simulink model "vtol50kg_linearization"  (R2024b)
settings: Solver=FixedStepAuto  StartTime=0.0  StopTime=10  FixedStep=5/1000  RelTol=1e-3
settings Model: DataDictionary=nextpilot_datadict.sldd  Creator=CETCA  LastModifiedBy=CETCA
settings DataIOCC: ExternalInput=getinputstruct(report8)  InitialState=getstatestruct(report8)  LoadExternalInput=on  LoadInitialState=on

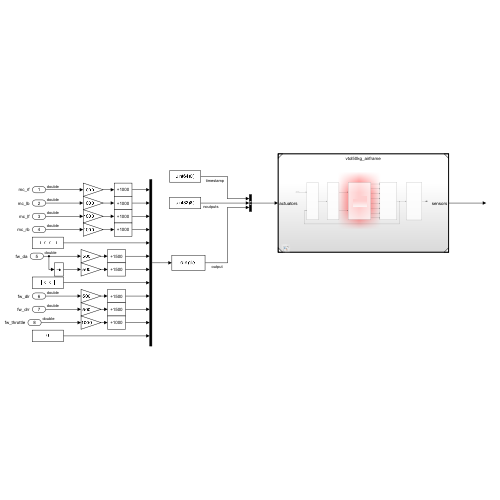
[thumbnail: Simulink's stored preview of the top-level diagram]
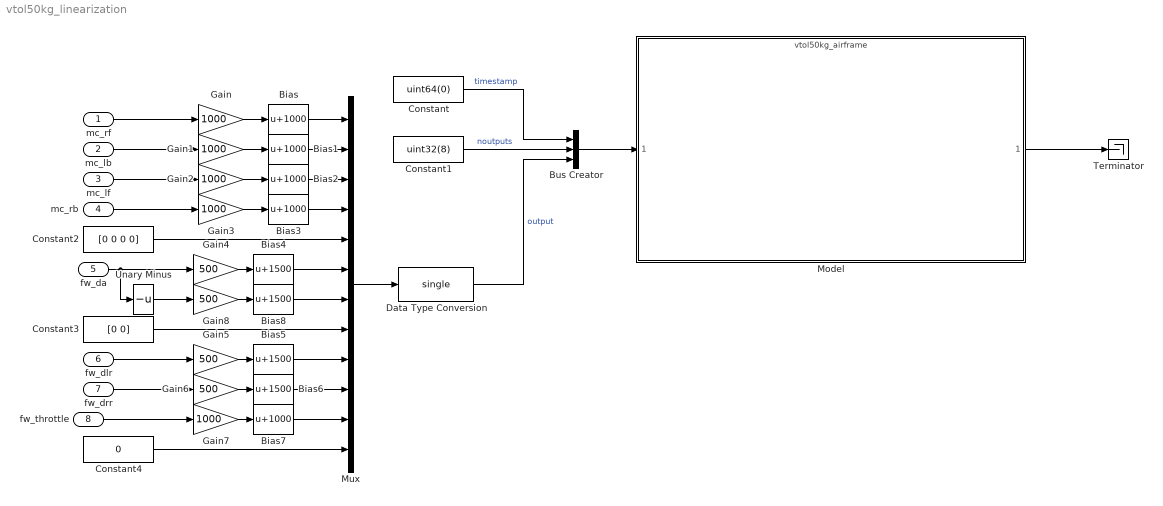
== system vtol50kg_linearization ==
  mc_rf : Inport  OutMin=0  OutMax=1  OutDataTypeStr=double
  mc_lb : Inport  Port=2  OutMin=0  OutMax=1  OutDataTypeStr=double
  mc_lf : Inport  Port=3  OutMin=0  OutMax=1  OutDataTypeStr=double
  mc_rb : Inport  Port=4  OutMin=0  OutMax=1  OutDataTypeStr=double
  fw_da : Inport  Port=5  OutMin=-1  OutMax=1  OutDataTypeStr=double
  fw_dlr : Inport  Port=6  OutMin=-1  OutMax=1  OutDataTypeStr=double
  fw_drr : Inport  Port=7  OutMin=-1  OutMax=1  OutDataTypeStr=double
  fw_throttle : Inport  Port=8  OutMin=0  OutMax=1  OutDataTypeStr=double
  Bias{,1..3,7} (5 alike) : Bias  Bias=1000  SaturateOnIntegerOverflow=off
  Bias{4..6,8} (4 alike) : Bias  Bias=1500  SaturateOnIntegerOverflow=off
  Bus Creator : BusCreator  Inputs=3
  Constant : Constant  Value=uint64(0)
  Constant1 : Constant  Value=uint32(8)
  Constant2 : Constant  Value=[0 0 0 0]
  Constant3 : Constant  Value=[0 0]
  Constant4 : Constant  Value=0
  Data Type Conversion : DataTypeConversion  OutDataTypeStr=single  SaturateOnIntegerOverflow=off  RndMeth=Floor
  Gain{,1..3,7} (5 alike) : Gain  Gain=1000
  Gain{4..6,8} (4 alike) : Gain  Gain=500
  Model : ModelReference  ModelNameDialog=vtol50kg_airframe.slx  SimulationMode=Normal  ModelReferenceVersion=5.112
  Mux : Mux  Inputs=12
  Terminator : Terminator
  Unary Minus : UnaryMinus
  wires:
  Bus Creator/1 -> Model/1
  Constant/1 -> Bus Creator/1  "timestamp"
  Constant1/1 -> Bus Creator/2  "noutputs"
  Mux/1 -> Data Type Conversion/1
  Data Type Conversion/1 -> Bus Creator/3  "output"
  Model/1 -> Terminator/1
  mc_lb/1 -> Gain1/1
  mc_lf/1 -> Gain2/1
  mc_rf/1 -> Gain/1
  mc_rb/1 -> Gain3/1
  Constant2/1 -> Mux/5
  fw_da/1 -> Unary Minus/1, Gain4/1
  Constant3/1 -> Mux/8
  fw_dlr/1 -> Gain5/1
  fw_drr/1 -> Gain6/1
  fw_throttle/1 -> Gain7/1
  Constant4/1 -> Mux/12
  Gain/1 -> Bias/1
  Bias/1 -> Mux/1
  Gain1/1 -> Bias1/1
  Bias1/1 -> Mux/2
  Gain2/1 -> Bias2/1
  Bias2/1 -> Mux/3
  Gain3/1 -> Bias3/1
  Bias3/1 -> Mux/4
  Gain4/1 -> Bias4/1
  Bias4/1 -> Mux/6
  Gain5/1 -> Bias5/1
  Bias5/1 -> Mux/9
  Gain6/1 -> Bias6/1
  Bias6/1 -> Mux/10
  Gain7/1 -> Bias7/1
  Bias7/1 -> Mux/11
  Unary Minus/1 -> Gain8/1
  Gain8/1 -> Bias8/1
  Bias8/1 -> Mux/7
